simulink model "ecg_modelo"  (Simulink 8.0)
settings: Solver=FixedStepDiscrete  StartTime=0.0  StopTime=10  FixedStep=Ts  RelTol=1e-3
values from neighbouring files (symbols this model uses):
  Ts = 0.1E-3    (= 0.0001)    [main.m]
libraries: commnoisgen2 x1
Description:
  | Real-Time Signal Generator
  | 
  | This demonstration shows how to produce an analog output signal using
  | Real-Time Windows Target. Because analog output typically requires
  | less configuration and is easier to connect than analog input, this demo
  | is a good start to your experiments with data acquisition boards. You can
  | verify the presence of the generated signal e.g. by connecting an
  | oscilloscope to the analog output pins of your data acquisition board.
  | 
  | How to run this demo:
  | 
  |   1. Open the Analog Output block and select your data acquisition board.
  |       If there's no board installed, install it using the Install new board button.
  |   2. Build the model using Tools -> Code Generation -> Build Model.
  |   3. Connect to the real-time code using Simulation -> Connect to target.
  |   4. Start the real-time execution using Simulation -> Start real-time code.
  | 
  | Note:
  | To run this demo, you must have a data acquisition board plugged into your computer.
settings Model: Creator=The MathWorks Inc.  LastModifiedBy=H243  ExtModeTrigType=signal  ExtModeTrigLevel=0.500000
settings DataIOCC: SignalLoggingSaveFormat=ModelDataLogs  SignalLoggingName=logsOut
settings OptimizationCC: InitFltsAndDblsToZero=on  EfficientMapNaN2IntZero=off
settings DebuggingCC: SignalResolutionControl=TryResolveAllWithWarning  SolverPrmCheckMsg=none  FcnCallInpInsideContextMsg=UseLocalSettings  StrictBusMsg=Warning
settings HardwareCC: ProdIntDivRoundTo=Zero  ProdEndianess=LittleEndian  ProdHWDeviceType=32-bit Real-Time Windows Target
settings RTWCC: SystemTargetFile=rtwin.tlc  TemplateMakefile=rtwin.tmf  Description=Real-Time Windows Target  ProcessScript=rtwin_make_rtw_hook
settings CodeAppCC: CustomSymbolStrType=$N$R$M_T  InternalIdentifier=Shortened
settings TargetCC: TargetLibSuffix=_rtwin.lib  TargetPreCompLibLocation=C:\Program Files\MATLAB\R2011a\toolbox\rtw\targets\rtwin\lib\win32  CodeReplacementLibrary=ANSI_C  IsPILTarget=off  EnableShiftOperators=on
settings CustomProperty: DataType=string

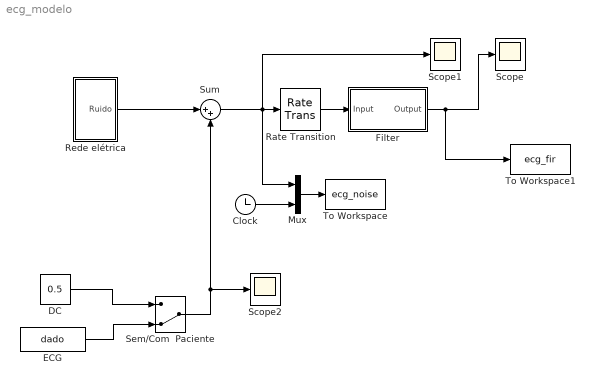
== system ecg_modelo ==
  Clock : Clock
  DC : Constant  Value=0.5
  ECG : FromWorkspace  VariableName=dado  SampleTime=Ts  Interpolate=off  OutputAfterFinalValue=Cyclic repetition
  Filter : Subsystem  Tag=FilterWizardSubSystem
      settings: ErrorFcn=dspFilterRealizedInBasicElemsAlgLoopErrFcnCallback
  Mux : Mux  Inputs=2
  Rate Transition : RateTransition  OutPortSampleTime=1E-2
  Rede elétrica : Subsystem
  Scope : Scope
      settings: TimeRange=1000  YMin=-0.11  YMax=0.11
  Scope1 : Scope
      settings: TimeRange=1000  YMin=-0.11  YMax=0.11
  Scope2 : Scope
      settings: TimeRange=1000  YMin=-0.11  YMax=0.11  SaveName=ScopeData2
  Sem/Com  Paciente : ManualSwitch  CurrentSetting=0
  Sum : Sum  Inputs=|++  SampleTime=Ts
  To Workspace : ToWorkspace  VariableName=ecg_noise  SampleTime=Ts
  To Workspace1 : ToWorkspace  VariableName=ecg_fir  SampleTime=1e-2
  wires:
  Sum/1 -> Rate Transition/1, Scope1/1, Mux/1
  Mux/1 -> To Workspace/1
  Clock/1 -> Mux/2
  ECG/1 -> Sem/Com  Paciente/2
  DC/1 -> Sem/Com  Paciente/1
  Sem/Com  Paciente/1 -> Scope2/1, Sum/2
  Rede elétrica/1(Ruido) -> Sum/1
  Rate Transition/1 -> Filter/1(Input)
  Filter/1(Output) -> To Workspace1/1, Scope/1

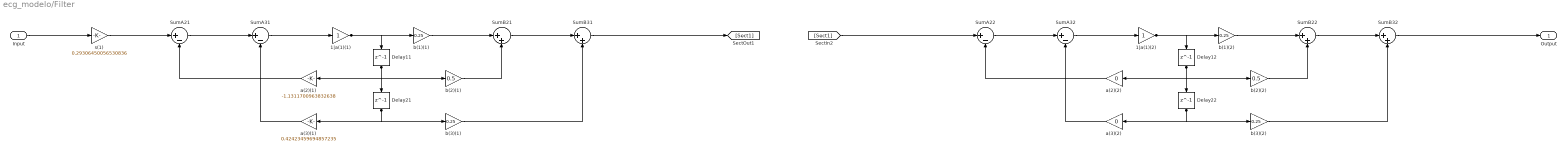
== system ecg_modelo/Filter ==
  Input : Inport
  1|a(1)(1) : Gain  ParamDataTypeStr=double  RndMeth=Nearest  SaturateOnIntegerOverflow=on  OutDataTypeStr=Inherit: Same as input
  1|a(1)(2) : Gain  ParamDataTypeStr=double  RndMeth=Nearest  SaturateOnIntegerOverflow=on  OutDataTypeStr=Inherit: Same as input
  Delay{11..12,21..22} (4 alike) : Delay  DelayLength=1  InitialCondition=0
  SumA{21..22,31..32} (4 alike) : Sum  Inputs=|+-  RndMeth=Nearest  SaturateOnIntegerOverflow=on  OutDataTypeStr=Inherit: Same as first input
  SumB{21..22,31..32} (4 alike) : Sum  Inputs=|++  RndMeth=Nearest  SaturateOnIntegerOverflow=on  OutDataTypeStr=Inherit: Same as first input
  a(2)(1) : Gain  Gain=-1.1311700963832638  ParamDataTypeStr=double  RndMeth=Nearest  SaturateOnIntegerOverflow=on  OutDataTypeStr=Inherit: Same as input
  a(2)(2) : Gain  Gain=0  ParamDataTypeStr=double  RndMeth=Nearest  SaturateOnIntegerOverflow=on  OutDataTypeStr=Inherit: Same as input
  a(3)(1) : Gain  Gain=0.42423459694857235  ParamDataTypeStr=double  RndMeth=Nearest  SaturateOnIntegerOverflow=on  OutDataTypeStr=Inherit: Same as input
  a(3)(2) : Gain  Gain=0  ParamDataTypeStr=double  RndMeth=Nearest  SaturateOnIntegerOverflow=on  OutDataTypeStr=Inherit: Same as input
  b(1)(1) : Gain  Gain=0.25  ParamDataTypeStr=double  RndMeth=Nearest  SaturateOnIntegerOverflow=on  OutDataTypeStr=Inherit: Same as input
  b(1)(2) : Gain  Gain=0.25  ParamDataTypeStr=double  RndMeth=Nearest  SaturateOnIntegerOverflow=on  OutDataTypeStr=Inherit: Same as input
  b(2)(1) : Gain  Gain=0.5  ParamDataTypeStr=double  RndMeth=Nearest  SaturateOnIntegerOverflow=on  OutDataTypeStr=Inherit: Same as input
  b(2)(2) : Gain  Gain=0.5  ParamDataTypeStr=double  RndMeth=Nearest  SaturateOnIntegerOverflow=on  OutDataTypeStr=Inherit: Same as input
  b(3)(1) : Gain  Gain=0.25  ParamDataTypeStr=double  RndMeth=Nearest  SaturateOnIntegerOverflow=on  OutDataTypeStr=Inherit: Same as input
  b(3)(2) : Gain  Gain=0.25  ParamDataTypeStr=double  RndMeth=Nearest  SaturateOnIntegerOverflow=on  OutDataTypeStr=Inherit: Same as input
  s(1) : Gain  Gain=0.29306450056530836  ParamDataTypeStr=double  RndMeth=Nearest  SaturateOnIntegerOverflow=on  OutDataTypeStr=Inherit: Same as input
  Output : Outport
  wires:
  Input/1 -> s(1)/1
  s(1)/1 -> SumA21/1
  SumA21/1 -> SumA31/1
  SumA31/1 -> 1|a(1)(1)/1
  1|a(1)(1)/1 -> b(1)(1)/1, Delay11/1
  b(1)(1)/1 -> SumB21/1
  SumB21/1 -> SumB31/1
  SumB31/1 -> [Sect1]
  a(2)(1)/1 -> SumA21/2
  Delay11/1 -> a(2)(1)/1, b(2)(1)/1, Delay21/1
  b(2)(1)/1 -> SumB21/2
  a(3)(1)/1 -> SumA31/2
  Delay21/1 -> a(3)(1)/1, b(3)(1)/1
  b(3)(1)/1 -> SumB31/2
  [Sect1] -> SumA22/1
  SumA22/1 -> SumA32/1
  SumA32/1 -> 1|a(1)(2)/1
  1|a(1)(2)/1 -> b(1)(2)/1, Delay12/1
  b(1)(2)/1 -> SumB22/1
  SumB22/1 -> SumB32/1
  SumB32/1 -> Output/1
  a(2)(2)/1 -> SumA22/2
  Delay12/1 -> a(2)(2)/1, b(2)(2)/1, Delay22/1
  b(2)(2)/1 -> SumB22/2
  a(3)(2)/1 -> SumA32/2
  Delay22/1 -> a(3)(2)/1, b(3)(2)/1
  b(3)(2)/1 -> SumB32/2

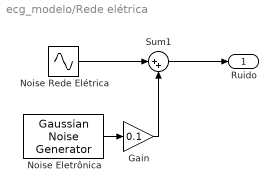
== system ecg_modelo/Rede elétrica ==
  Gain : Gain  Gain=0.1
  Noise Eletrônica : commnoisgen2/Gaussian Noise Generator  m=0  d=1  s=41  Ts=Ts  frameBased=off  sampPerFrame=1  orient=off  outDataType=double
  Noise Rede Elétrica : Sin  Frequency=60*2*pi  Samples=60  SampleTime=Ts
  Sum1 : Sum  Inputs=|++  SampleTime=Ts
  Ruido : Outport
  wires:
  Noise Rede Elétrica/1 -> Sum1/1
  Sum1/1 -> Ruido/1
  Noise Eletrônica/1 -> Gain/1
  Gain/1 -> Sum1/2
